simulink model "PMSM_FOC_Model_Chapter3"  (R2021a)
settings: Solver=FixedStepDiscrete  StartTime=0.0  StopTime=10.0  RelTol=1e-3
settings Model: Creator=Wu  LastModifiedBy=Wu

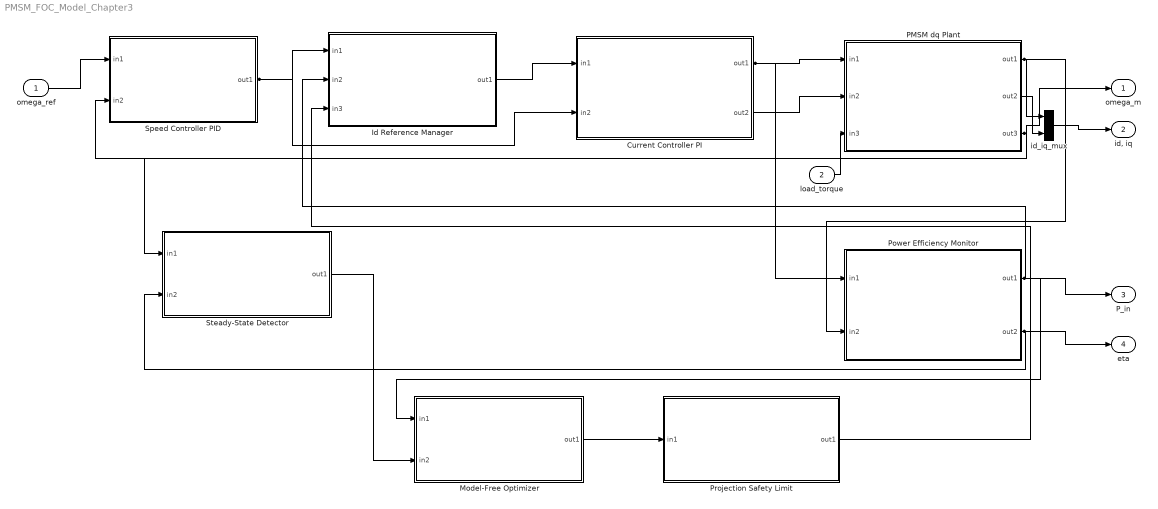
== system PMSM_FOC_Model_Chapter3 ==
  omega_ref : Inport
  load_torque : Inport  Port=2
  Current Controller PI : Subsystem
      mask Display: disp('Current Controller PI')
  Id Reference Manager : Subsystem
      mask Display: disp('Id Reference Manager')
  Model-Free Optimizer : Subsystem
      mask Display: disp('Model-Free Optimizer')
  PMSM dq Plant : Subsystem
      mask Display: disp('PMSM dq Plant')
  Power Efficiency Monitor : Subsystem
      mask Display: disp('Power Efficiency Monitor')
  Projection Safety Limit : Subsystem
      mask Display: disp('Projection / Safety Limit')
  Speed Controller PID : Subsystem
      mask Display: disp('Speed Controller PID')
  Steady-State Detector : Subsystem
      mask Display: disp('Steady-State Detector')
  id_iq_mux : Mux  Inputs=2
  omega_m : Outport
  "id, iq" : Outport  Port=2
  P_in : Outport  Port=3
  eta : Outport  Port=4
  wires:
  omega_ref/1 -> Speed Controller PID/1(in1)
  Speed Controller PID/1(out1) -> Id Reference Manager/1(in1), Current Controller PI/2(in2)
  Id Reference Manager/1(out1) -> Current Controller PI/1(in1)
  Current Controller PI/1(out1) -> PMSM dq Plant/1(in1), Power Efficiency Monitor/1(in1)
  Current Controller PI/2(out2) -> PMSM dq Plant/2(in2)
  load_torque/1 -> PMSM dq Plant/3(in3)
  PMSM dq Plant/3(out3) -> Speed Controller PID/2(in2), Steady-State Detector/1(in1), omega_m/1
  PMSM dq Plant/1(out1) -> Power Efficiency Monitor/2(in2), id_iq_mux/1
  Power Efficiency Monitor/2(out2) -> Steady-State Detector/2(in2), eta/1
  Power Efficiency Monitor/1(out1) -> Id Reference Manager/2(in2), Model-Free Optimizer/1(in1), P_in/1
  Steady-State Detector/1(out1) -> Model-Free Optimizer/2(in2)
  Model-Free Optimizer/1(out1) -> Projection Safety Limit/1(in1)
  Projection Safety Limit/1(out1) -> Id Reference Manager/3(in3)
  PMSM dq Plant/2(out2) -> id_iq_mux/2
  id_iq_mux/1 -> "id, iq"/1

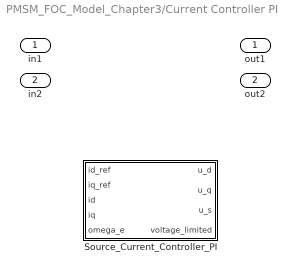
== system PMSM_FOC_Model_Chapter3/Current Controller PI ==
  in1 : Inport
  in2 : Inport  Port=2
  Source_Current_Controller_PI : Subsystem
  out1 : Outport
  out2 : Outport  Port=2

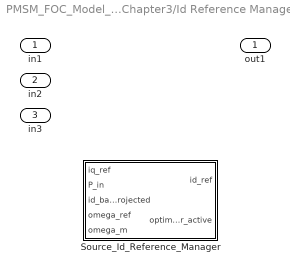
== system PMSM_FOC_Model_Chapter3/Id Reference Manager ==
  in1 : Inport
  in2 : Inport  Port=2
  in3 : Inport  Port=3
  Source_Id_Reference_Manager : Subsystem
  out1 : Outport

== system PMSM_FOC_Model_Chapter3/Model-Free Optimizer ==
  in1 : Inport
  in2 : Inport  Port=2
  Source_ModelFree_Optimizer : Subsystem
  out1 : Outport

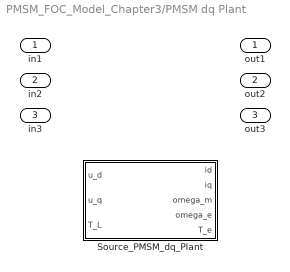
== system PMSM_FOC_Model_Chapter3/PMSM dq Plant ==
  in1 : Inport
  in2 : Inport  Port=2
  in3 : Inport  Port=3
  Source_PMSM_dq_Plant : Subsystem
  out1 : Outport
  out2 : Outport  Port=2
  out3 : Outport  Port=3

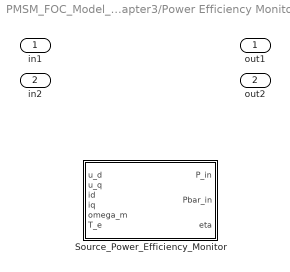
== system PMSM_FOC_Model_Chapter3/Power Efficiency Monitor ==
  in1 : Inport
  in2 : Inport  Port=2
  Source_Power_Efficiency_Monitor : Subsystem
  out1 : Outport
  out2 : Outport  Port=2

== system PMSM_FOC_Model_Chapter3/Projection Safety Limit ==
  in1 : Inport
  Source_Projection_Omega : Subsystem
  out1 : Outport

== system PMSM_FOC_Model_Chapter3/Speed Controller PID ==
  in1 : Inport
  in2 : Inport  Port=2
  Source_Speed_Controller_PID : Subsystem
  out1 : Outport

== system PMSM_FOC_Model_Chapter3/Steady-State Detector ==
  in1 : Inport
  in2 : Inport  Port=2
  Source_SteadyState_Detector : Subsystem
  out1 : Outport

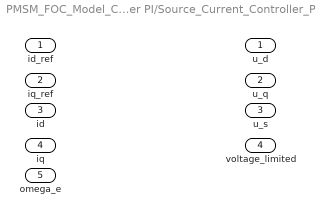
== system PMSM_FOC_Model_Chapter3/Current Controller PI/Source_Current_Controller_PI ==
  id_ref : Inport
  iq_ref : Inport  Port=2
  id : Inport  Port=3
  iq : Inport  Port=4
  omega_e : Inport  Port=5
  u_d : Outport
  u_q : Outport  Port=2
  u_s : Outport  Port=3
  voltage_limited : Outport  Port=4

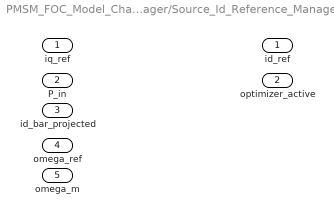
== system PMSM_FOC_Model_Chapter3/Id Reference Manager/Source_Id_Reference_Manager ==
  iq_ref : Inport
  P_in : Inport  Port=2
  id_bar_projected : Inport  Port=3
  omega_ref : Inport  Port=4
  omega_m : Inport  Port=5
  id_ref : Outport
  optimizer_active : Outport  Port=2

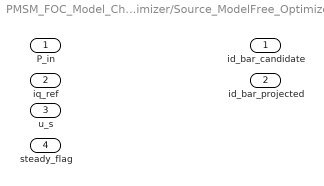
== system PMSM_FOC_Model_Chapter3/Model-Free Optimizer/Source_ModelFree_Optimizer ==
  P_in : Inport
  iq_ref : Inport  Port=2
  u_s : Inport  Port=3
  steady_flag : Inport  Port=4
  id_bar_candidate : Outport
  id_bar_projected : Outport  Port=2

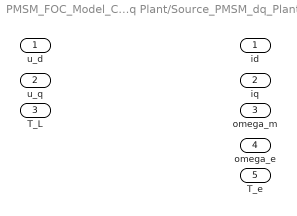
== system PMSM_FOC_Model_Chapter3/PMSM dq Plant/Source_PMSM_dq_Plant ==
  u_d : Inport
  u_q : Inport  Port=2
  T_L : Inport  Port=3
  id : Outport
  iq : Outport  Port=2
  omega_m : Outport  Port=3
  omega_e : Outport  Port=4
  T_e : Outport  Port=5

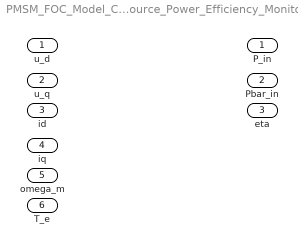
== system PMSM_FOC_Model_Chapter3/Power Efficiency Monitor/Source_Power_Efficiency_Monitor ==
  u_d : Inport
  u_q : Inport  Port=2
  id : Inport  Port=3
  iq : Inport  Port=4
  omega_m : Inport  Port=5
  T_e : Inport  Port=6
  P_in : Outport
  Pbar_in : Outport  Port=2
  eta : Outport  Port=3

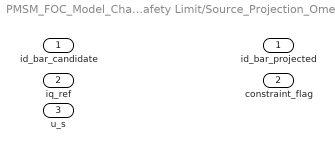
== system PMSM_FOC_Model_Chapter3/Projection Safety Limit/Source_Projection_Omega ==
  id_bar_candidate : Inport
  iq_ref : Inport  Port=2
  u_s : Inport  Port=3
  id_bar_projected : Outport
  constraint_flag : Outport  Port=2

== system PMSM_FOC_Model_Chapter3/Speed Controller PID/Source_Speed_Controller_PID ==
  omega_ref : Inport
  omega_m : Inport  Port=2
  iq_ref : Outport
  speed_error : Outport  Port=2

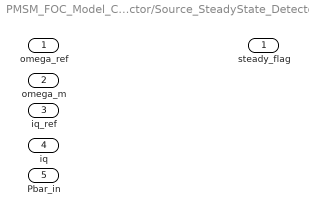
== system PMSM_FOC_Model_Chapter3/Steady-State Detector/Source_SteadyState_Detector ==
  omega_ref : Inport
  omega_m : Inport  Port=2
  iq_ref : Inport  Port=3
  iq : Inport  Port=4
  Pbar_in : Inport  Port=5
  steady_flag : Outport
